simulink model "s385"  (Simulink 8.2)
settings: Solver=ode45  StartTime=0.0  StopTime=inf  RelTol=1e-3
values from neighbouring files (symbols this model uses):
  den = sym2poly(s*(M1*(M2+m)*s^2 + (c*s+K)*(M1+M2+m)))    [PIDPDSolution.m]    (also in el_vars.mat = [51000 490 9800000 0]; elevator_variables.mat = [51000 490 9800000 0])
  num = sym2poly(c*s + K)    [PIDPDSolution.m]    (also in el_vars.mat = [1 20000]; elevator_variables.mat = [1 20000])
libraries: simulink x2, vrlib x2
settings Model: Creator=Trina  LastModifiedBy=Nate
settings OptimizationCC: InitFltsAndDblsToZero=on

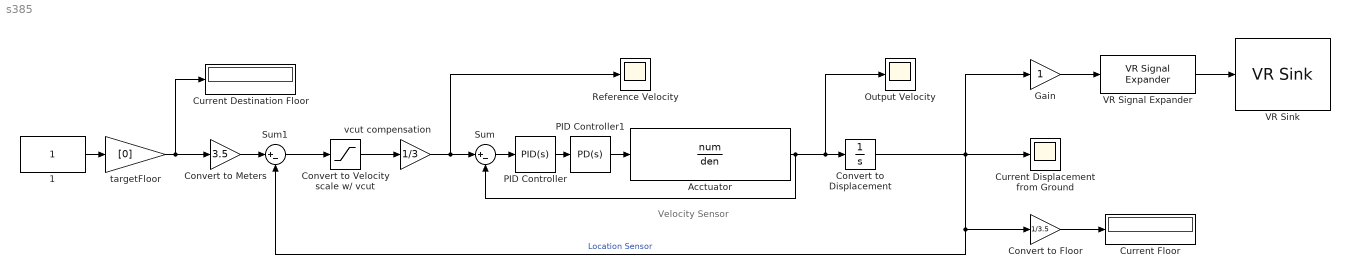
== system s385 ==
  note: Velocity Sensor
  1 : Constant
  Acctuator : TransferFcn  Numerator=num  Denominator=den
  Convert to Velocity scale w/ vcut : Saturate  UpperLimit=3  LowerLimit=-3
  Convert to Meters : Gain  Gain=3.5
  Convert to Displacement : Integrator
  Convert to Floor : Gain  Gain=1/3.5
  Current Destination Floor : Display
  Current Displacement from Ground : Scope
      settings: YMin=17.491  YMax=17.51
  Current Floor : Display
  Gain : Gain
  Output Velocity : Scope
      settings: YMin=-0.00045  YMax=-5e-05
  PID Controller : simulink/Continuous/PID Controller  Controller=PID  TimeDomain=Continuous-time  SampleTime=1  IntegratorMethod=Forward Euler  FilterMethod=Forward Euler  Form=Parallel  P=5  I=24  D=1  N=100  InitialConditionSource=internal  InitialConditionForIntegrator=0  InitialConditionForFilter=0  ExternalReset=none  LimitOutput=off  UpperSaturationLimit=inf  LowerSaturationLimit=-inf  LinearizeAsGain=on  AntiWindupMode=none  Kb=1  TrackingMode=off  Kt=1  PParamMin=[]  PParamMax=[]  IParamMin=[]  IParamMax=[]  DParamMin=[]  DParamMax=[]  NParamMin=[]  NParamMax=[]  KbParamMin=[]  KbParamMax=[]  KtParamMin=[]  KtParamMax=[]  POutMin=[]  POutMax=[]  IOutMin=[]  IOutMax=[]  DOutMin=[]  DOutMax=[]  NOutMin=[]  NOutMax=[]  KbOutMin=[]  KbOutMax=[]  KtOutMin=[]  KtOutMax=[]  IntegratorOutMin=[]  IntegratorOutMax=[]  FilterOutMin=[]  FilterOutMax=[]  SumOutMin=[]  SumOutMax=[]  SumI1OutMin=[]  SumI1OutMax=[]  SumI2OutMin=[]  SumI2OutMax=[]  SumI3OutMin=[]  SumI3OutMax=[]  SumDOutMin=[]  SumDOutMax=[]  SaturationOutMin=[]  SaturationOutMax=[]  IntegratorContinuousStateAttributes=''  IntegratorStateMustResolveToSignalObject=off  IntegratorRTWStateStorageClass=Auto  FilterContinuousStateAttributes=''  FilterStateMustResolveToSignalObject=off  FilterRTWStateStorageClass=Auto
  PID Controller1 : simulink/Continuous/PID Controller  Controller=PD  TimeDomain=Continuous-time  SampleTime=1  IntegratorMethod=Forward Euler  FilterMethod=Forward Euler  Form=Parallel  P=1  I=1  D=9  N=100  InitialConditionSource=internal  InitialConditionForIntegrator=0  InitialConditionForFilter=0  ExternalReset=none  LimitOutput=off  UpperSaturationLimit=inf  LowerSaturationLimit=-inf  LinearizeAsGain=on  AntiWindupMode=none  Kb=1  TrackingMode=off  Kt=1  PParamMin=[]  PParamMax=[]  IParamMin=[]  IParamMax=[]  DParamMin=[]  DParamMax=[]  NParamMin=[]  NParamMax=[]  KbParamMin=[]  KbParamMax=[]  KtParamMin=[]  KtParamMax=[]  POutMin=[]  POutMax=[]  IOutMin=[]  IOutMax=[]  DOutMin=[]  DOutMax=[]  NOutMin=[]  NOutMax=[]  KbOutMin=[]  KbOutMax=[]  KtOutMin=[]  KtOutMax=[]  IntegratorOutMin=[]  IntegratorOutMax=[]  FilterOutMin=[]  FilterOutMax=[]  SumOutMin=[]  SumOutMax=[]  SumI1OutMin=[]  SumI1OutMax=[]  SumI2OutMin=[]  SumI2OutMax=[]  SumI3OutMin=[]  SumI3OutMax=[]  SumDOutMin=[]  SumDOutMax=[]  SaturationOutMin=[]  SaturationOutMax=[]  IntegratorContinuousStateAttributes=''  IntegratorStateMustResolveToSignalObject=off  IntegratorRTWStateStorageClass=Auto  FilterContinuousStateAttributes=''  FilterStateMustResolveToSignalObject=off  FilterRTWStateStorageClass=Auto
  Reference Velocity : Scope
      settings: YMin=-1e-013  YMax=1.2e-012  SaveName=ScopeData2
  Sum : Sum  Inputs=|+-
  Sum1 : Sum  Inputs=|+-
  VR Signal Expander : vrlib/VR Signal Expander  outwidth=3  outidx=[2]
  VR Sink : vrlib/VR Sink  InstantiateOnLoad=on  SampleTime=0.1  ViewEnable=on  RemoteChange=off  RemoteView=on  FieldsWritten=elevator.translation.3.1.double  WorldFileName=s385.WRL  AutoView=off  VideoDimensions=[]  AllowVariableSize=off
  targetFloor : Gain  Gain=[0]
  vcut compensation : Gain  Gain=1/3
  wires:
  Sum/1 -> PID Controller/1
  Gain/1 -> VR Signal Expander/1
  VR Signal Expander/1 -> VR Sink/1
  Convert to Floor/1 -> Current Floor/1
  Acctuator/1 -> Convert to Displacement/1, Output Velocity/1, Sum/2
  1/1 -> targetFloor/1
  targetFloor/1 -> Convert to Meters/1, Current Destination Floor/1
  Convert to Meters/1 -> Sum1/1
  Convert to Velocity scale w/ vcut/1 -> vcut compensation/1
  vcut compensation/1 -> Sum/1, Reference Velocity/1
  Sum1/1 -> Convert to Velocity scale w/ vcut/1
  Convert to Displacement/1 -> Current Displacement from Ground/1, Sum1/2, Convert to Floor/1, Gain/1  "Location Sensor"
  PID Controller/1 -> PID Controller1/1
  PID Controller1/1 -> Acctuator/1
